simulink model "sim_cf95a"  (Simulink 6.2)
settings: Solver=ode45  StartTime=0.0  StopTime=10.0  MaxStep=1.e-3  RelTol=1e-3
undefined symbols (not defined in the file or in its folder): dGh, dGm, dK, nGh, nGm, nK, T, tau
libraries: simulink x1
settings Model: LastModifiedBy=Administrator
settings OptimizationCC: BlockReduction=off  BooleanDataType=off  InlineInvariantSignals=on
settings HardwareCC: TargetUnknown=on

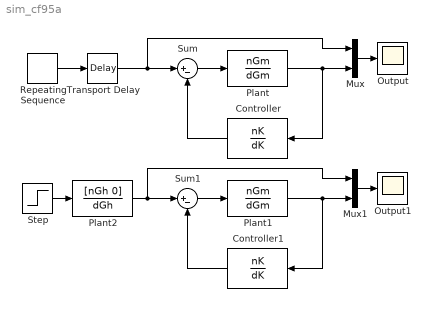
== system sim_cf95a ==
  Controller : DiscreteTransferFcn  Orientation=left  Numerator=nK  Denominator=dK  SampleTime=T
  Controller1 : DiscreteTransferFcn  Orientation=left  Numerator=nK  Denominator=dK  SampleTime=T
  Mux : Mux  Inputs=2
  Mux1 : Mux  Inputs=2
  Output : Scope
      settings: TimeRange=10  YMin=-1  YMax=2  SaveName=y  DataFormat=Array
  Output1 : Scope
      settings: TimeRange=10  YMin=-1  YMax=2  SaveName=yApp  DataFormat=Array
  Plant : TransferFcn  Numerator=nGm  Denominator=dGm
  Plant1 : TransferFcn  Numerator=nGm  Denominator=dGm
  Plant2 : TransferFcn  Numerator=[nGh 0]  Denominator=dGh
  Repeating Sequence : simulink/Sources/Repeating Sequence  rep_seq_t=[0 0.5 1 1.5 2 10]  rep_seq_y="[0 1 2  1 0 0]"
  Step : Step  Time=tau  SampleTime=0
  Sum : Sum  Inputs=|+-  SaturateOnIntegerOverflow=on  InputSameDT=on
  Sum1 : Sum  Inputs=|+-  SaturateOnIntegerOverflow=on  InputSameDT=on
  Transport Delay : TransportDelay  DelayTime=tau  BufferSize=10000  PadeOrder=4
  wires:
  Repeating Sequence/1 -> Transport Delay/1
  Transport Delay/1 -> Sum/1, Mux/1
  Sum/1 -> Plant/1
  Controller/1 -> Sum/2
  Plant/1 -> Controller/1, Mux/2
  Mux/1 -> Output/1
  Plant2/1 -> Mux1/1, Sum1/1
  Sum1/1 -> Plant1/1
  Controller1/1 -> Sum1/2
  Plant1/1 -> Mux1/2, Controller1/1
  Mux1/1 -> Output1/1
  Step/1 -> Plant2/1
